simulink model "V_S"  (R2023b)
settings: Solver=VariableStepAuto  StartTime=0.0  StopTime=t(end)  RelTol=1e-3
settings Model: Creator=franc  LastModifiedBy=franc
settings DebuggingCC: AlgebraicLoopMsg=none

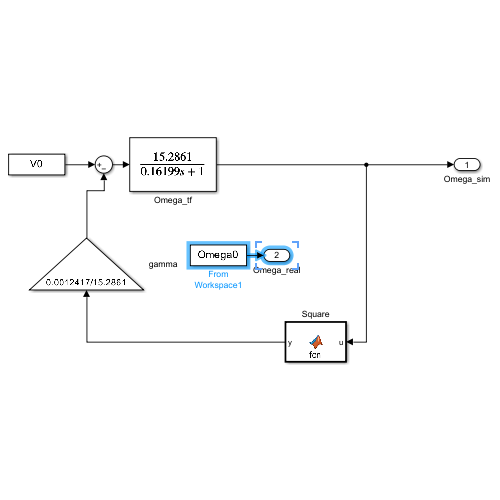
[thumbnail: Simulink's stored preview of the top-level diagram]
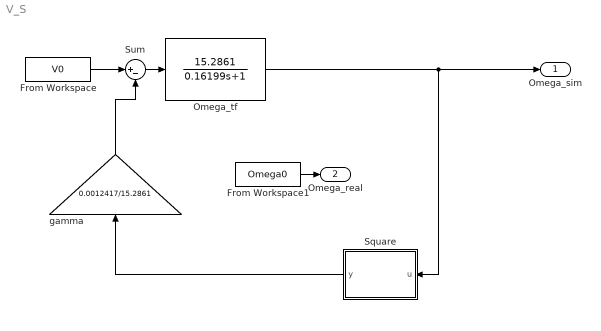
== system V_S ==
  From Workspace : FromWorkspace  VariableName=V0
  From Workspace1 : FromWorkspace  VariableName=Omega0  SampleTime=t(2)-t(1)
  Omega_tf : TransferFcn  Numerator=15.2861  Denominator=[0.16199 1]
  Square : MATLAB Function  TreatAsAtomicUnit=on
  Sum : Sum  Inputs=|+-
  gamma : Gain  Gain=0.0012417/15.2861
  Omega_sim : Outport
  Omega_real : Outport  Port=2
  wires:
  From Workspace/1 -> Sum/1
  gamma/1 -> Sum/2
  Omega_tf/1 -> Square/1(u), Omega_sim/1
  From Workspace1/1 -> Omega_real/1
  Sum/1 -> Omega_tf/1
  Square/1(y) -> gamma/1

== matlab function V_S/Square ==
  data: u input; y output
function y = fcn(u)
y=u^2*sign(u);
